simulink model "exp4_p1"  (R2018a)
settings: Solver=VariableStepAuto  StartTime=0.0  StopTime=10.0  RelTol=1e-3
settings Model: Creator=Administrator  LastModifiedBy=Administrator

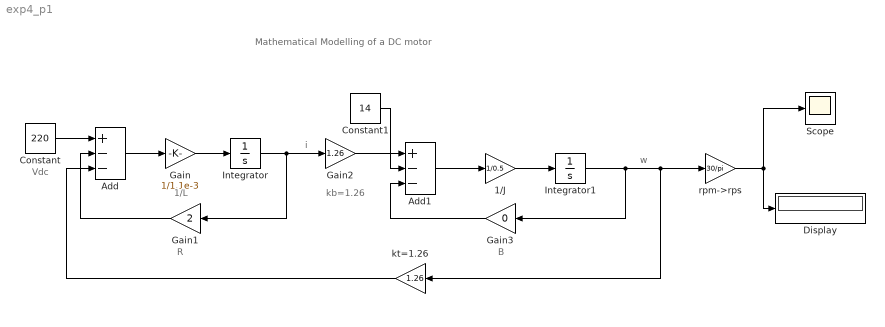
== system exp4_p1 ==
  note: Mathematical Modelling of a DC motor
  note: Vdc
  note: w
  note: B
  note: kb=1.26
  note: i
  note: R
  note: 1/L
  "1/J " : Gain  Gain=1/0.5
  Add : Sum  Inputs=+--
  Add1 : Sum  Inputs=+--
  Constant : Constant  Value=220
  Constant1 : Constant  Value=14
  Display : Display
  Gain : Gain  Gain=1/1.1e-3
  Gain1 : Gain  Gain=2
  Gain2 : Gain  Gain=1.26
  Gain3 : Gain  Gain=0
  Integrator : Integrator
  Integrator1 : Integrator
  Scope : Scope
  "kt=1.26 " : Gain  Gain=1.26
  rpm->rps : Gain  Gain=30/pi
  wires:
  Constant/1 -> Add/1
  Add/1 -> Gain/1
  Gain/1 -> Integrator/1
  Gain1/1 -> Add/2
  Integrator/1 -> Gain2/1, Gain1/1
  Gain2/1 -> Add1/1
  Add1/1 -> "1/J "/1
  "1/J "/1 -> Integrator1/1
  "kt=1.26 "/1 -> Add/3
  Integrator1/1 -> Gain3/1, rpm->rps/1, "kt=1.26 "/1
  Gain3/1 -> Add1/3
  Constant1/1 -> Add1/2
  rpm->rps/1 -> Scope/1, Display/1
